simulink model "EJERCICIO_5"  (R2024b)
settings: Solver=VariableStepAuto  StartTime=0.0  StopTime=10  RelTol=1e-3
values from neighbouring files (symbols this model uses):
  ts = 0.00001    (= 1e-05)    [script.m]
libraries: spsSeriesRLCBranchLib x3, spsCurrentMeasurementLib x1, spsDCVoltageSourceLib x1, spsVoltageMeasurementLib x1, spspowerguiLib x1
settings Model: Creator=Antonio  LastModifiedBy=pacoc
settings DataIOCC: ReturnWorkspaceOutputs=off
settings RTWCC: GPUComputeCapability=3.5

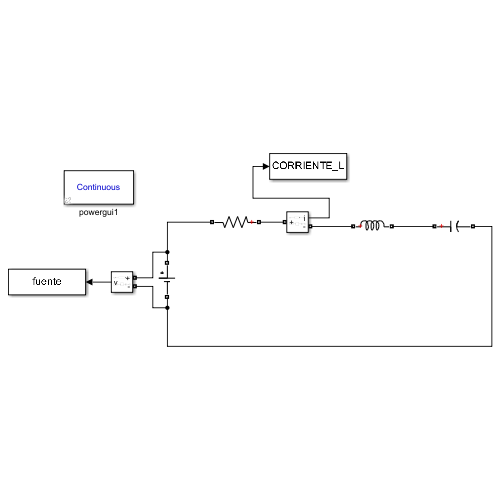
[thumbnail: Simulink's stored preview of the top-level diagram]
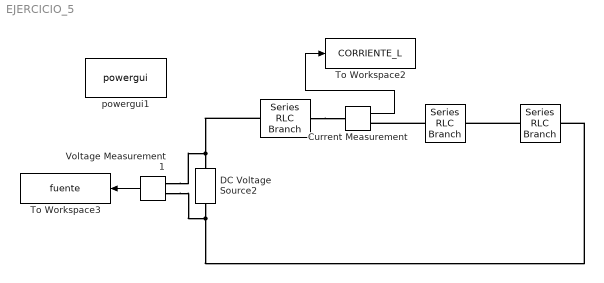
== system EJERCICIO_5 ==
  "  " : spsSeriesRLCBranchLib/Series RLC Branch  LConnTagsString=__new0  RConnTagsString=__new0  BranchType=R  Resistance=400  Inductance=0.03  SetiL0=on  InitialCurrent=0  Capacitance=0.000220  Setx0=on  InitialVoltage=9  Measurements=None
  "           " : spsSeriesRLCBranchLib/Series RLC Branch  LConnTagsString=__new0  RConnTagsString=__new0  BranchType=C  Resistance=330  Inductance=0.03  SetiL0=on  InitialCurrent=0  Capacitance=0.000010  Setx0=on  InitialVoltage=0  Measurements=None
  "                                  " : spsSeriesRLCBranchLib/Series RLC Branch  LConnTagsString=__new0  RConnTagsString=__new0  BranchType=L  Resistance=330  Inductance=1  SetiL0=on  InitialCurrent=0  Capacitance=0.000220  Setx0=on  InitialVoltage=0  Measurements=None
  Current Measurement : spsCurrentMeasurementLib/Current Measurement  PhasorSimulation=off  OutputType=Complex  PSBequivalent=0
  DC Voltage Source2 : spsDCVoltageSourceLib/DC Voltage Source  Amplitude=15  Measurements=Voltage
  To Workspace2 : ToWorkspace  VariableName=CORRIENTE_L  SampleTime=ts
  To Workspace3 : ToWorkspace  VariableName=fuente  SampleTime=ts
  Voltage Measurement1 : spsVoltageMeasurementLib/Voltage Measurement  PhasorSimulation=off  OutputType=Complex  PSBequivalent=0
  powergui1 : spspowerguiLib/powergui  Priority=1  SimulationMode=Continuous  SampleTime=50e-6  frequency=50  Iterations=50  frequencyindice=0  Pbase=100e6  ErrMax=1e-4  UnitsV=kV  UnitsW=MW  buscounter=0  FunctionMessages=off  echomessages=off  EnableUseOfTLC=off  CurrentSourceSwitches=off  DisableSnubberDevices=off  DisableRonSwitches=off  DisableVfSwitches=off  DisplayEquations=off  AutomaticDiscreteSolvers=off  SolverType=Tustin/Backward Euler (TBE)  Interpol=off  ExternalGateDelay=off  methode=off  Ts=100  x0status=blocks  SPID=on  SwTol=0  HookPort=off  NonlinearTolerance=1e-4  nMaxIteration=100  ContinueOnMaxIteration=off  RestoreLinks=warning  ResistiveCurrentMeasurement=off  Frange=[0:2:500]  Ylog=off  Xlog=on  ShowGrid=off  save=off  variable=ZData  structure=0  ZoomFFT=off  StartTime=0.0  cycles=1  DisplayStyle=1  fundamental=60  FreqAxis=off  MaxFrequency=1000  frequencyindicesteady=1  RmsSteady=1  display=off
  wires:
  Current Measurement/1 -> To Workspace2/1
  Voltage Measurement1/1 -> To Workspace3/1
  connections:
  "                                  "/LConn1 -- Current Measurement/RConn1
  "  "/LConn1 -- Current Measurement/LConn1
  "  "/RConn1 -- Voltage Measurement1/LConn1 -- DC Voltage Source2/RConn1
  "           "/LConn1 -- "                                  "/RConn1
  "           "/RConn1 -- Voltage Measurement1/LConn2 -- DC Voltage Source2/LConn1
